simulink model "TF_exmpl"  (R2021a)
settings: Solver=VariableStepAuto  StartTime=0.0  StopTime=10  RelTol=1e-3
settings Model: Creator=Panok  LastModifiedBy=Panok

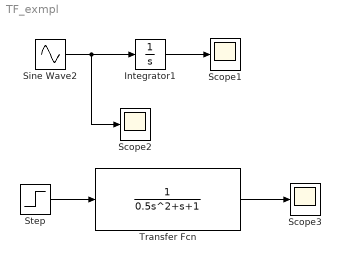
== system TF_exmpl ==
  Integrator1 : Integrator  ZeroCross=off
  Scope1 : Scope
  Scope2 : Scope
  Scope3 : Scope
  Sine Wave2 : Sin  Frequency=2*pi*10  SampleTime=0
  Step : Step  SampleTime=0
  Transfer Fcn : TransferFcn  Denominator=[0.5 1 1]
  wires:
  Sine Wave2/1 -> Scope2/1, Integrator1/1
  Integrator1/1 -> Scope1/1
  Step/1 -> Transfer Fcn/1
  Transfer Fcn/1 -> Scope3/1
